simulink model "OFFSET_3"  (R2022b)
settings: Solver=FixedStepDiscrete  StartTime=0  StopTime=duration  FixedStep=0.1  RelTol=1e-3
settings Model: Creator=Carlo_TUM  LastModifiedBy=Carlo_TUM
settings DataIOCC: ReturnWorkspaceOutputs=off  ReturnWorkspaceOutputsName=off
settings OptimizationCC: DefaultParameterBehavior=Inlined  EnhancedBackFolding=on  PassReuseOutputArgsAs=Individual arguments  OptimizeBlockOrder=speed  DifferentSizesBufferReuse=on  OptimizationCustomize=off  EfficientTunableParamExpr=on
settings DebuggingCC: ParameterTunabilityLossMsg=error
settings SFSimCC: MATLABDynamicMemAlloc=off
settings RTWCC: Description=Embedded Coder  SystemTargetFile=ert.tlc  TemplateMakefile=ert_default_tmf
settings CodeAppCC: ForceParamTrailComments=on  IgnoreCustomStorageClasses=off  OperatorAnnotations=on  SimulinkDataObjDesc=on  SFDataObjDesc=on  InsertBlockDesc=on
settings ERTTargetCC: TargetLangStandard=C99 (ISO)  GenerateSampleERTMain=on  InlinedParameterPlacement=NonHierarchical  ERTCustomFileTemplate=example_file_process.tlc

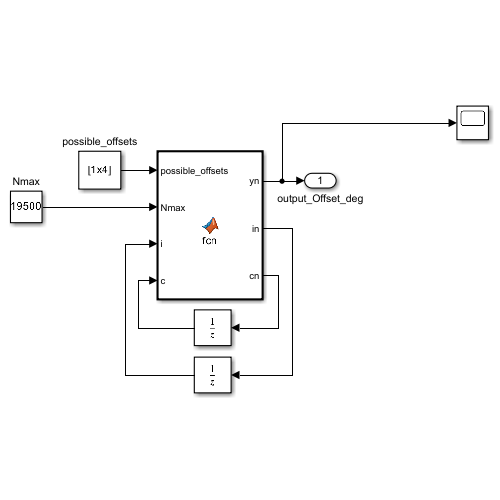
[thumbnail: Simulink's stored preview of the top-level diagram]
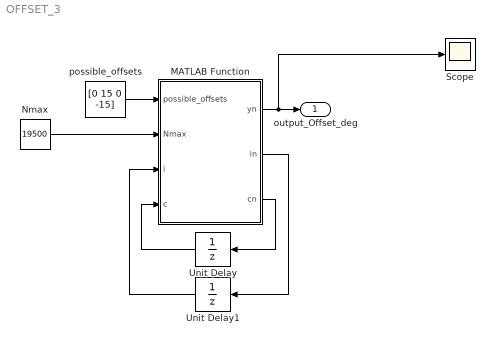
== system OFFSET_3 ==
  MATLAB Function : MATLAB Function  TreatAsAtomicUnit=on
  Nmax : Constant  Value=19500
  Scope : Scope
  Unit Delay : UnitDelay  SampleTime=0.1  HasFrameUpgradeWarning=on
  Unit Delay1 : UnitDelay  SampleTime=0.1  HasFrameUpgradeWarning=on
  possible_offsets : Constant  Value=[0 15 0 -15]
  output_Offset_deg : Outport  VectorParamsAs1DForOutWhenUnconnected=off
  wires:
  Unit Delay1/1 -> MATLAB Function/3(i)
  MATLAB Function/1(yn) -> Scope/1, output_Offset_deg/1
  Unit Delay/1 -> MATLAB Function/4(c)
  Nmax/1 -> MATLAB Function/2(Nmax)
  MATLAB Function/3(cn) -> Unit Delay/1
  possible_offsets/1 -> MATLAB Function/1(possible_offsets)
  MATLAB Function/2(in) -> Unit Delay1/1

== matlab function OFFSET_3/MATLAB Function ==
  data: possible_offsets input; Nmax input; yn output; i input; c input; in output; cn output
function [yn,in,cn] = fcn(possible_offsets,Nmax,i,c)

% Nmax = 39000; % 65*60/.1;
Noff = numel(possible_offsets);

if Noff<1
    yn = 0;
    in = 0;
    cn = 0;
    return
end

cn = mod(c + 1,Nmax);

if cn, in = mod(i,Noff);
else, in = mod(i+1,Noff);
end

yn = possible_offsets(in+1);
